simulink model "model_a"  (R2024b)
settings: Solver=ode4  StartTime=0.0  StopTime=simTime  FixedStep=sample_time  RelTol=1e-3
values from neighbouring files (symbols this model uses):
  b = 1    [init.m]    (also in init_a.m; init_b.m; init_ca.m; init_cb.m)
  gamma = 6    [init.m]    (also in init_a.m = 1; init_b.m = 0.05*2^(i-1)/2; init_ca.m = 5; init_cb.m = 1)
  sineAmp = 1    [init_a.m]    (also in init_b.m; init_ca.m = 0.1*2^(i-1)/2; init_cb.m; init_d.m = 1000)
settings Model: Creator=kemal  LastModifiedBy=akdal

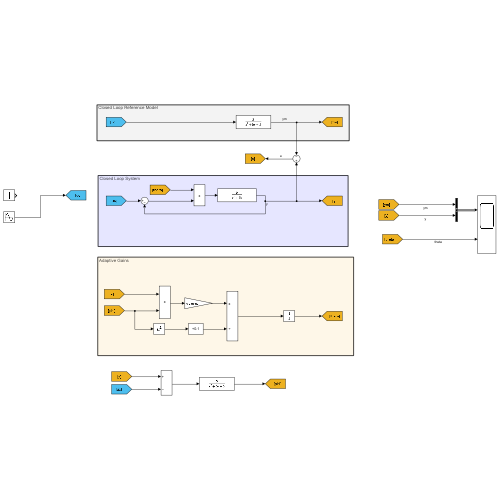
[thumbnail: Simulink's stored preview of the top-level diagram]
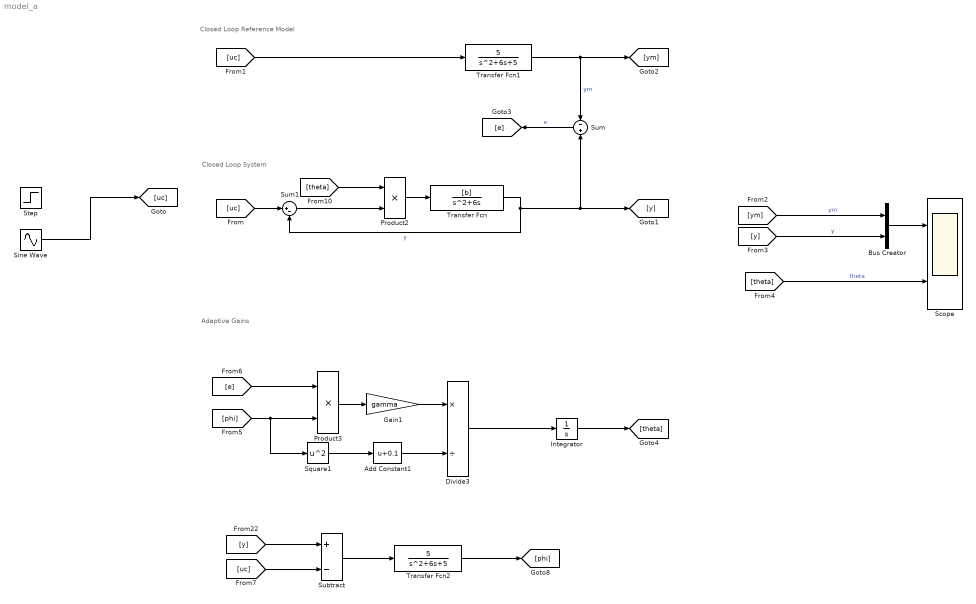
== system model_a ==
  note: Closed Loop Reference Model
  note: Adaptive Gains
  note: Closed Loop System
  Add Constant1 : Bias  Bias=0.1  SaturateOnIntegerOverflow=off
  Bus Creator : BusCreator  Inputs=2
  Divide3 : Product  Inputs=*/
  Gain1 : Gain  Gain=gamma
  Integrator : Integrator
  Product2 : Product
  Product3 : Product
  Scope : Scope  NumInputPorts=2
  Sine Wave : Sin  Amplitude=sineAmp  Frequency=2*pi/5  SampleTime=0
  Square1 : Math  Operator=square
  Step : Step  SampleTime=0
  Subtract : Sum  Inputs=+-
  Sum : Sum  Inputs=-+
  Sum1 : Sum  Inputs=|+-
  Transfer Fcn : TransferFcn  Numerator=[b]  Denominator=[1 6 0]
  Transfer Fcn1 : TransferFcn  Numerator=[5]  Denominator=[1 6 5]
  Transfer Fcn2 : TransferFcn  Numerator=[5]  Denominator=[1 6 5]
  wires:
  [uc] -> Transfer Fcn1/1
  Transfer Fcn1/1 -> [ym], Sum/1  "ym"
  Transfer Fcn/1 -> Sum/2, [y], Sum1/2  "y"
  Sine Wave/1 -> [uc]
  [ym] -> Bus Creator/1  "ym"
  [y] -> Bus Creator/2  "y"
  Bus Creator/1 -> Scope/1
  [theta] -> Scope/2  "theta"
  [uc] -> Sum1/1
  Sum/1 -> [e]  "e"
  Integrator/1 -> [theta]
  Divide3/1 -> Integrator/1
  [theta] -> Product2/1
  Add Constant1/1 -> Divide3/2
  Square1/1 -> Add Constant1/1
  [phi] -> Square1/1, Product3/2
  [e] -> Product3/1
  Product3/1 -> Gain1/1
  Gain1/1 -> Divide3/1
  [y] -> Subtract/1
  [uc] -> Subtract/2
  Subtract/1 -> Transfer Fcn2/1
  Sum1/1 -> Product2/2
  Product2/1 -> Transfer Fcn/1
  Transfer Fcn2/1 -> [phi]
